simulink model "enabsubs_org"  (Simulink 10.0)
settings: Solver=ode45  StartTime=0.0  StopTime=10  MaxStep=0.1  RelTol=1e-3  AbsTol=1e-6
Description:
  | Advanced Enabled Subsystems
  | 
  | This model shows what happens when a sine wave is fed into an enabled
  |  subsystem. The four subsystems in the model contain integrators, either discrete or
  |  continuous as described by the Subsystem name. After running the simulation, the two
  |  scopes show the results for the discrete enabled subsystems (top scope) and
  |  continuous enabled subsystems (bottom scope.)
  | 
  | Each Scope shows the output for all combinations of where the states or outputs of the
  | enabled subsystem are either held or reset when the subsystem is disabled. The colors
  | on the scope correspond to the following state and output configuration.
  | 
  | Yellow: Reset states; Held outputs
  | 
  | Purple: Reset states; Reset outputs
  | 
  | Cyan: Held states; Held outputs
  | 
  | Red: Held states; Reset outputs
settings Model: Creator=The MathWorks, Inc.  LastModifiedBy=bhisma  ExtModeTrigMode=oneshot  ExtModeArmWhenConnect=off  ExtModeAutoUpdateStatusClock=off
settings SolverCC: AutoScaleAbsTol=off
settings DataIOCC: ExternalInput=[]  InitialState=[]  ReturnWorkspaceOutputs=on
settings OptimizationCC: BlockReduction=off  BooleanDataType=off  ExpressionDepthLimit=2147483647  InitFltsAndDblsToZero=on
settings DebuggingCC: SaveWithParameterizedLinksMsg=none  UnderspecifiedInitializationDetection=Simplified  MergeDetectMultiDrivingBlocksExec=error  SignalResolutionControl=TryResolveAllWithWarning  MultiTaskDSMMsg=warning  MultiTaskCondExecSysMsg=none  FcnCallInpInsideContextMsg=warning  AllowSymbolicDim=off  StateNameClashWarn=warning
settings HardwareCC: TargetUnknown=on
settings GRTTargetCC: TargetFcnLib=ansi_tfl_tmw.mat  GeneratePreprocessorConditionals=Disable all
settings ConfigComp: CovExternalEMLEnable=off

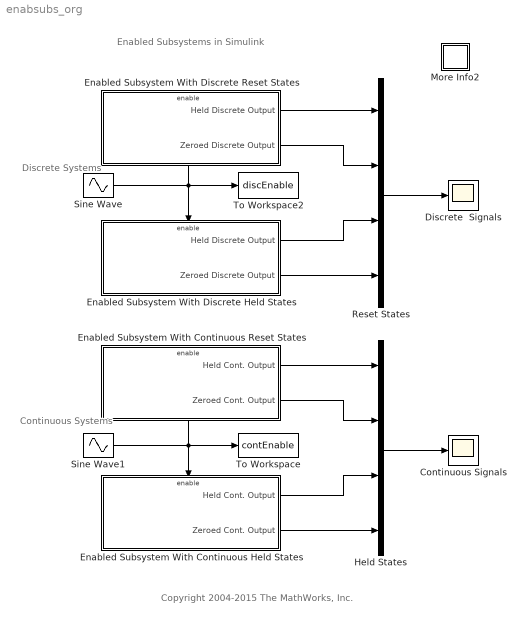
== system enabsubs_org ==
  note: Enabled Subsystems in Simulink
  note: Discrete
      | Systems
  note: Continuous
      | Systems
  note: Copyright 2004-2015 The MathWorks, Inc.
  Continuous Signals : Scope
  Discrete  Signals : Scope
  Enabled Subsystem With Continuous Held States : Subsystem
  Enabled Subsystem With Continuous Reset States : Subsystem
  Enabled Subsystem With Discrete Held States : Subsystem
  Enabled Subsystem With Discrete Reset States : Subsystem
  Held States : Mux
  More Info2 : Subsystem
      settings: OpenFcn=showdemo(bdroot(gcs))
      mask Display: disp('?')
  Reset States : Mux
  Sine Wave : Sin  Frequency=pi  SampleTime=0.1
  Sine Wave1 : Sin  Frequency=pi  SampleTime=0
  To Workspace : ToWorkspace  VariableName=contEnable  SampleTime=-1
  To Workspace2 : ToWorkspace  VariableName=discEnable  SampleTime=-1
  wires:
  Enabled Subsystem With Discrete Held States/1(Held Discrete Output) -> Reset States/3
  Enabled Subsystem With Discrete Held States/2(Zeroed Discrete Output) -> Reset States/4
  Enabled Subsystem With Discrete Reset States/1(Held Discrete Output) -> Reset States/1
  Enabled Subsystem With Discrete Reset States/2(Zeroed Discrete Output) -> Reset States/2
  Sine Wave/1 -> Enabled Subsystem With Discrete Held States/Enable, Enabled Subsystem With Discrete Reset States/Enable, To Workspace2/1
  Reset States/1 -> Discrete  Signals/1
  Enabled Subsystem With Continuous Reset States/1(Held Cont. Output) -> Held States/1
  Enabled Subsystem With Continuous Reset States/2(Zeroed Cont. Output) -> Held States/2
  Enabled Subsystem With Continuous Held States/1(Held Cont. Output) -> Held States/3
  Enabled Subsystem With Continuous Held States/2(Zeroed Cont. Output) -> Held States/4
  Sine Wave1/1 -> To Workspace/1, Enabled Subsystem With Continuous Reset States/Enable, Enabled Subsystem With Continuous Held States/Enable
  Held States/1 -> Continuous Signals/1

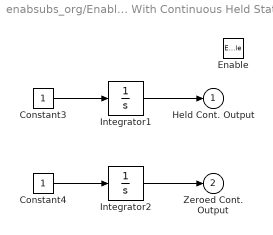
== system enabsubs_org/Enabled Subsystem With Continuous Held States ==
  Enable : EnablePort  PropagateVarSize=During execution
  Constant3 : Constant
  Constant4 : Constant
  Integrator1 : Integrator
  Integrator2 : Integrator
  Held Cont. Output : Outport  InitialOutput=0  VectorParamsAs1DForOutWhenUnconnected=off
  Zeroed Cont. Output : Outport  Port=2  OutputWhenDisabled=reset  InitialOutput=0  VectorParamsAs1DForOutWhenUnconnected=off
  wires:
  Constant3/1 -> Integrator1/1
  Integrator1/1 -> Held Cont. Output/1
  Constant4/1 -> Integrator2/1
  Integrator2/1 -> Zeroed Cont. Output/1

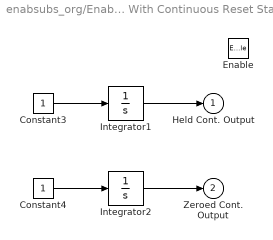
== system enabsubs_org/Enabled Subsystem With Continuous Reset States ==
  Enable : EnablePort  StatesWhenEnabling=reset  PropagateVarSize=During execution
  Constant3 : Constant
  Constant4 : Constant
  Integrator1 : Integrator
  Integrator2 : Integrator
  Held Cont. Output : Outport  InitialOutput=0  VectorParamsAs1DForOutWhenUnconnected=off
  Zeroed Cont. Output : Outport  Port=2  OutputWhenDisabled=reset  InitialOutput=0  VectorParamsAs1DForOutWhenUnconnected=off
  wires:
  Constant3/1 -> Integrator1/1
  Integrator1/1 -> Held Cont. Output/1
  Constant4/1 -> Integrator2/1
  Integrator2/1 -> Zeroed Cont. Output/1

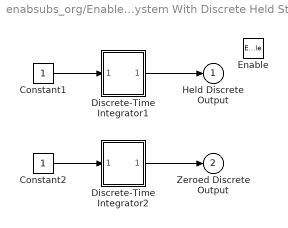
== system enabsubs_org/Enabled Subsystem With Discrete Held States ==
  Enable : EnablePort  PropagateVarSize=During execution
  Constant1 : Constant
  Constant2 : Constant
  Discrete-Time Integrator1 : Subsystem  mask(Discrete-Time Integrator){X0=0, Ts=.1}
      mask prompts: X0 "Initial Condition:"; Ts "Sample Time:"
      mask help: Discrete-Time Integrator:
      mask Help: Implements a zeroth order discrete\nintegration using a gain, a sum, and\na unit delay. Inputs may be scalar\nor vector.\n
      mask Display: dpoly(Ts,[1 -1],'z')
  Discrete-Time Integrator2 : Subsystem  mask(Discrete-Time Integrator){X0=0, Ts=.1}
      mask prompts: X0 "Initial Condition:"; Ts "Sample Time:"
      mask help: Discrete-Time Integrator:
      mask Help: Implements a zeroth order discrete\nintegration using a gain, a sum, and\na unit delay. Inputs may be scalar\nor vector.\n
      mask Display: dpoly(Ts,[1 -1],'z')
  Held Discrete Output : Outport  InitialOutput=0  VectorParamsAs1DForOutWhenUnconnected=off
  Zeroed Discrete Output : Outport  Port=2  OutputWhenDisabled=reset  InitialOutput=0  VectorParamsAs1DForOutWhenUnconnected=off
  wires:
  Discrete-Time Integrator2/1(out_1) -> Zeroed Discrete Output/1
  Constant2/1 -> Discrete-Time Integrator2/1(in_1)
  Discrete-Time Integrator1/1(out_1) -> Held Discrete Output/1
  Constant1/1 -> Discrete-Time Integrator1/1(in_1)

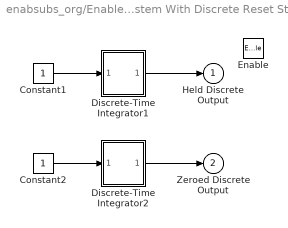
== system enabsubs_org/Enabled Subsystem With Discrete Reset States ==
  Enable : EnablePort  StatesWhenEnabling=reset  PropagateVarSize=During execution
  Constant1 : Constant
  Constant2 : Constant
  Discrete-Time Integrator1 : Subsystem  mask(Discrete-Time Integrator){X0=0, Ts=.1}
      mask prompts: X0 "Initial Condition:"; Ts "Sample Time:"
      mask help: Discrete-Time Integrator:
      mask Help: Implements a zeroth order discrete\nintegration using a gain, a sum, and\na unit delay. Inputs may be scalar\nor vector.\n
      mask Display: dpoly(Ts,[1 -1],'z')
  Discrete-Time Integrator2 : Subsystem  mask(Discrete-Time Integrator){X0=0, Ts=.1}
      mask prompts: X0 "Initial Condition:"; Ts "Sample Time:"
      mask help: Discrete-Time Integrator:
      mask Help: Implements a zeroth order discrete\nintegration using a gain, a sum, and\na unit delay. Inputs may be scalar\nor vector.\n
      mask Display: dpoly(Ts,[1 -1],'z')
  Held Discrete Output : Outport  InitialOutput=0  VectorParamsAs1DForOutWhenUnconnected=off
  Zeroed Discrete Output : Outport  Port=2  OutputWhenDisabled=reset  InitialOutput=0  VectorParamsAs1DForOutWhenUnconnected=off
  wires:
  Discrete-Time Integrator2/1(out_1) -> Zeroed Discrete Output/1
  Constant2/1 -> Discrete-Time Integrator2/1(in_1)
  Discrete-Time Integrator1/1(out_1) -> Held Discrete Output/1
  Constant1/1 -> Discrete-Time Integrator1/1(in_1)

== system enabsubs_org/More Info2 ==

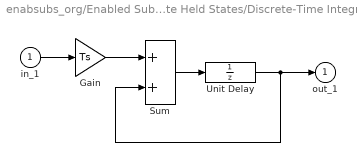
== system enabsubs_org/Enabled Subsystem With Discrete Held States/Discrete-Time Integrator1 ==
  in_1 : Inport
  Gain : Gain  Gain=Ts  SaturateOnIntegerOverflow=on  OutDataTypeStr=Inherit: Same as input  ParamDataTypeStr=Inherit: Same as input
  Sum : Sum  SaturateOnIntegerOverflow=on  InputSameDT=on  OutDataTypeStr=Inherit: Same as first input
  Unit Delay : UnitDelay  InitialCondition=X0  SampleTime=Ts  HasFrameUpgradeWarning=on
  out_1 : Outport  InitialOutput=0  VectorParamsAs1DForOutWhenUnconnected=off
  wires:
  Unit Delay/1 -> out_1/1, Sum/2
  Sum/1 -> Unit Delay/1
  in_1/1 -> Gain/1
  Gain/1 -> Sum/1

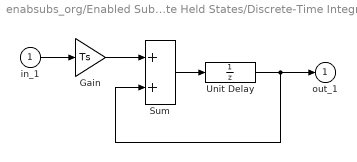
== system enabsubs_org/Enabled Subsystem With Discrete Held States/Discrete-Time Integrator2 ==
  in_1 : Inport
  Gain : Gain  Gain=Ts  SaturateOnIntegerOverflow=on  OutDataTypeStr=Inherit: Same as input  ParamDataTypeStr=Inherit: Same as input
  Sum : Sum  SaturateOnIntegerOverflow=on  InputSameDT=on  OutDataTypeStr=Inherit: Same as first input
  Unit Delay : UnitDelay  InitialCondition=X0  SampleTime=Ts  HasFrameUpgradeWarning=on
  out_1 : Outport  InitialOutput=0  VectorParamsAs1DForOutWhenUnconnected=off
  wires:
  Unit Delay/1 -> Sum/2, out_1/1
  Sum/1 -> Unit Delay/1
  in_1/1 -> Gain/1
  Gain/1 -> Sum/1

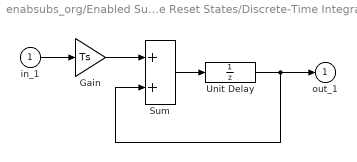
== system enabsubs_org/Enabled Subsystem With Discrete Reset States/Discrete-Time Integrator1 ==
  in_1 : Inport
  Gain : Gain  Gain=Ts  SaturateOnIntegerOverflow=on  OutDataTypeStr=Inherit: Same as input  ParamDataTypeStr=Inherit: Same as input
  Sum : Sum  SaturateOnIntegerOverflow=on  InputSameDT=on  OutDataTypeStr=Inherit: Same as first input
  Unit Delay : UnitDelay  InitialCondition=X0  SampleTime=Ts  HasFrameUpgradeWarning=on
  out_1 : Outport  InitialOutput=0  VectorParamsAs1DForOutWhenUnconnected=off
  wires:
  Unit Delay/1 -> Sum/2, out_1/1
  Sum/1 -> Unit Delay/1
  in_1/1 -> Gain/1
  Gain/1 -> Sum/1

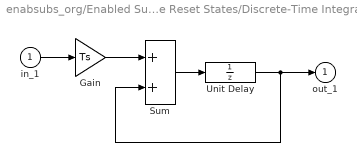
== system enabsubs_org/Enabled Subsystem With Discrete Reset States/Discrete-Time Integrator2 ==
  in_1 : Inport
  Gain : Gain  Gain=Ts  SaturateOnIntegerOverflow=on  OutDataTypeStr=Inherit: Same as input  ParamDataTypeStr=Inherit: Same as input
  Sum : Sum  SaturateOnIntegerOverflow=on  InputSameDT=on  OutDataTypeStr=Inherit: Same as first input
  Unit Delay : UnitDelay  InitialCondition=X0  SampleTime=Ts  HasFrameUpgradeWarning=on
  out_1 : Outport  InitialOutput=0  VectorParamsAs1DForOutWhenUnconnected=off
  wires:
  Unit Delay/1 -> out_1/1, Sum/2
  Sum/1 -> Unit Delay/1
  in_1/1 -> Gain/1
  Gain/1 -> Sum/1
